simulink subsystem "MR_Azimuth_model"  (R2025a)
settings: Solver=VariableStepAuto  StartTime=0.0  StopTime=10.0  RelTol=1e-3
settings Model: Creator=Admin  LastModifiedBy=Admin

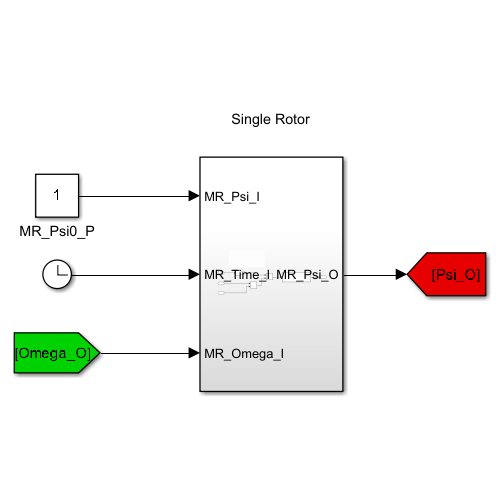
[thumbnail: Simulink's stored preview of the top-level diagram]
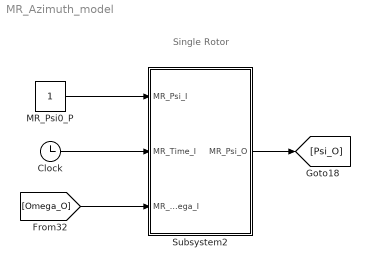
== system MR_Azimuth_model ==
  note: Single Rotor
  Clock : Clock
  MR_Psi0_P : Constant
  Subsystem2 : Subsystem
  wires:
  Subsystem2/1(MR_Psi_O) -> [Psi_O]
  Clock/1 -> Subsystem2/2(MR_Time_I)
  MR_Psi0_P/1 -> Subsystem2/1(MR_Psi_I)
  [Omega_O] -> Subsystem2/3(MR_Omega_I)

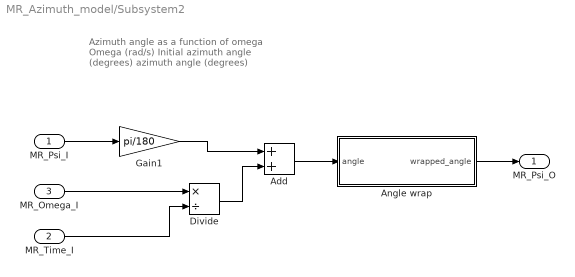
== system MR_Azimuth_model/Subsystem2 ==
  note: Azimuth angle as a function of omega
      | Omega (rad/s)
      | Initial azimuth angle (degrees)
      |
      | azimuth angle (degrees)
  MR_Psi_I : Inport
  MR_Time_I : Inport  Port=2
  MR_Omega_I : Inport  Port=3
  Add : Sum
  Angle wrap : MATLAB Function  TreatAsAtomicUnit=on
  Divide : Product  Inputs=*/
  Gain1 : Gain  Gain=pi/180
  MR_Psi_O : Outport
  wires:
  MR_Omega_I/1 -> Divide/1
  MR_Time_I/1 -> Divide/2
  Divide/1 -> Add/2
  MR_Psi_I/1 -> Gain1/1
  Gain1/1 -> Add/1
  Add/1 -> Angle wrap/1(angle)
  Angle wrap/1(wrapped_angle) -> MR_Psi_O/1

== matlab function MR_Azimuth_model/Subsystem2/Angle wrap ==
  data: angle input; wrapped_angle output
function wrapped_angle = angle_wrap(angle)
while angle >= 360
    angle = angle - 360;
end
while angle < 0
    angle = angle + 360;
end
wrapped_angle = angle;
